simulink model "forerunner_sim_replacement"  (R2016b)
settings: Solver=FixedStepAuto  StartTime=0.0  StopTime=duration  FixedStep=ts  RelTol=1e-3
PreLoadFcn:
  | forerunner_init
undefined symbols (not defined in the file): DiscIntNeverNeededParam, G, G_pitch, G_roll, G_yaw, h, initialEuler, initialPos, LLPV_Filter, P, Q, QC_mpc_rule, qc_update, R, s, S, sd, sdd, t_mpc, tmax, traj_res, UGV_init
libraries: simulink x5
settings Model: sldv_blockreplacement_configurable_lib=forerunner_sim_rt_lib  Creator=Misi  LastModifiedBy=Misi
settings DataIOCC: ReturnWorkspaceOutputs=on
settings DebuggingCC: ArtificialAlgebraicLoopMsg=none
settings SFSimCC: SimUseLocalCustomCode=on
settings RTWCC: RTWUseLocalCustomCode=on

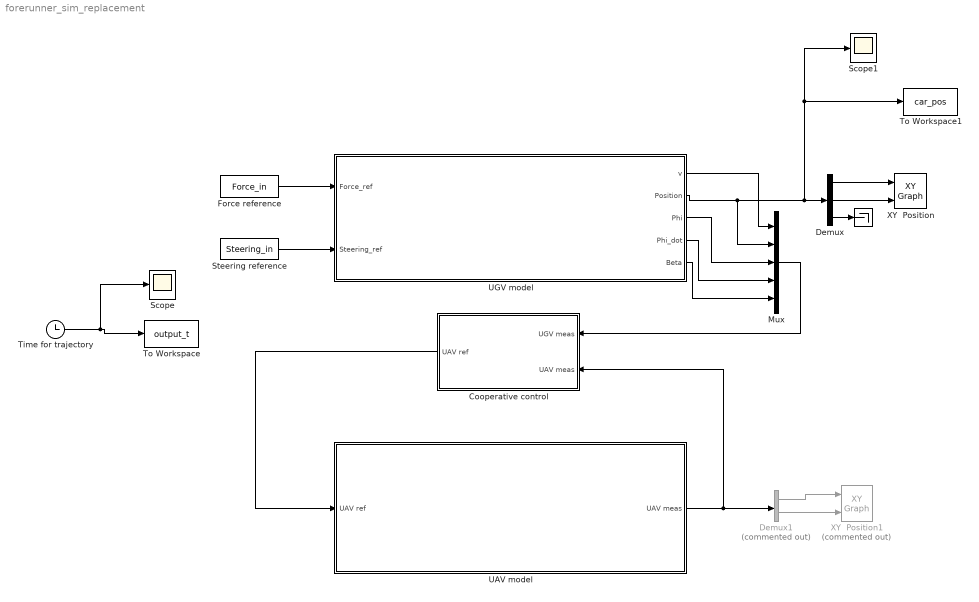
== system forerunner_sim_replacement ==
  " " : Terminator
  Cooperative control : Subsystem
  Demux : Demux  Outputs=3
  Demux1 : Demux  Commented=on  Outputs=2
  "Force reference " : FromWorkspace  VariableName=Force_in  SampleTime=0
  Mux : Mux  Inputs=5
  Scope : Scope
  Scope1 : Scope
  Steering reference : FromWorkspace  VariableName=Steering_in  SampleTime=0
  Time for trajectory : Clock
  To Workspace : ToWorkspace  VariableName=output_t  SampleTime=-1
  To Workspace1 : ToWorkspace  VariableName=car_pos  SampleTime=-1
  UAV model : Subsystem
  UGV model : Subsystem  TreatAsAtomicUnit=on  mask(Sldv ModelReference(Model name:UGV) Replacement){ModelName=UGV, ParameterArgumentNames=, ParameterArgumentValues=, SimulationMode=Normal}
      mask help: Replacement for the Model Reference block that references the model UGV. If Model arguments are specified on the Model Reference block, then they will appear in the mask parameters.
  XY 	Position : simulink/Sinks/XY Graph  xmin=-20  xmax=20  ymin=-20  ymax=20  st=-1
  XY 	Position1 : simulink/Sinks/XY Graph  Commented=on  xmin=-20  xmax=20  ymin=-20  ymax=20  st=-1
  wires:
  "Force reference "/1 -> UGV model/1(Force_ref)
  Steering reference/1 -> UGV model/2(Steering_ref)
  UGV model/2(Position) -> Mux/2, Scope1/1, To Workspace1/1, Demux/1
  Demux/1 -> XY 	Position/1
  Demux/2 -> XY 	Position/2
  UGV model/1(v) -> Mux/1
  UGV model/3(Phi) -> Mux/3
  UGV model/4(Phi_dot) -> Mux/4
  Mux/1 -> Cooperative control/1(UGV meas)
  UAV model/1(UAV meas) -> Cooperative control/2(UAV meas), Demux1/1
  Cooperative control/1(UAV ref) -> UAV model/1(UAV ref)
  Time for trajectory/1 -> Scope/1, To Workspace/1
  Demux/3 -> " "/1
  UGV model/5(Beta) -> Mux/5
  Demux1/1 -> XY 	Position1/1
  Demux1/2 -> XY 	Position1/2

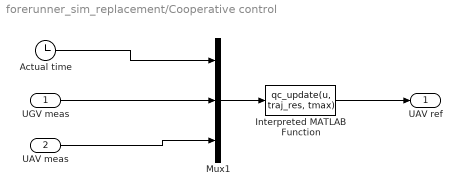
== system forerunner_sim_replacement/Cooperative control ==
  UGV meas : Inport
  UAV meas : Inport  Port=2
  Actual time : Clock
  Interpreted MATLAB Function : MATLABFcn  MATLABFcn=qc_update(u, traj_res, tmax)
  Mux1 : Mux  Inputs=3
  UAV ref : Outport
  wires:
  Interpreted MATLAB Function/1 -> UAV ref/1
  Mux1/1 -> Interpreted MATLAB Function/1
  Actual time/1 -> Mux1/1
  UGV meas/1 -> Mux1/2
  UAV meas/1 -> Mux1/3

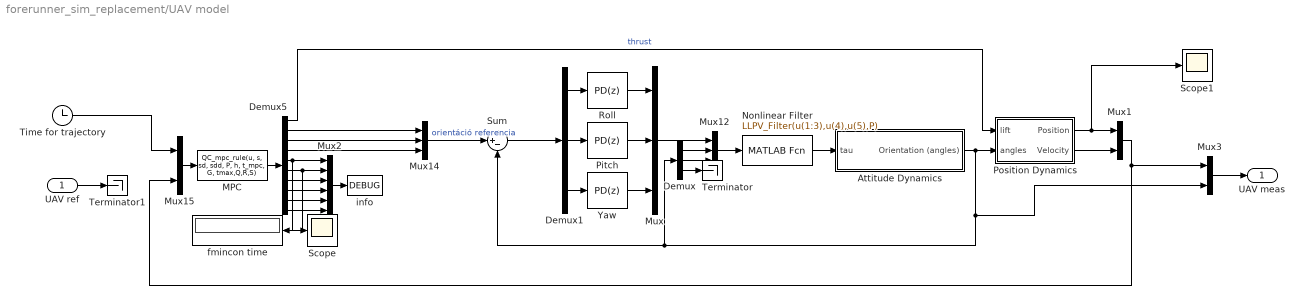
== system forerunner_sim_replacement/UAV model ==
  UAV ref : Inport
  Attitude Dynamics : Subsystem
  Demux : Demux  Outputs=3
  Demux1 : Demux  Outputs=3
  Demux5 : Demux  Outputs=10
  MPC : MATLABFcn  MATLABFcn=QC_mpc_rule(u, s, sd, sdd, P, h, t_mpc, G, tmax,Q,R,S)  OutputDimensions=10
  Mux : Mux  Inputs=3
  Mux1 : Mux  Inputs=2
  Mux12 : Mux  Inputs=3
  Mux14 : Mux  Inputs=3
  Mux15 : Mux  Inputs=2
  Mux2 : Mux  Inputs=6
  Mux3 : Mux  Inputs=2
  Nonlinear Filter : MATLABFcn  MATLABFcn=LLPV_Filter(u(1:3),u(4),u(5),P)  OutputDimensions=3
  Pitch : simulink/Continuous/PID Controller  Controller=PD  TimeDomain=Discrete-time  SampleTime=-1  IntegratorMethod=Forward Euler  FilterMethod=Forward Euler  Form=Parallel  UseFilter=on  ControllerParametersSource=internal  P=G_pitch.Kp  I=1  D=G_pitch.Kd  N=1/G_pitch.Tf  InitialConditionSource=internal  InitialConditionForIntegrator=0  InitialConditionForFilter=0  ExternalReset=none  LimitOutput=off  UpperSaturationLimit=inf  LowerSaturationLimit=-inf  LinearizeAsGain=on  AntiWindupMode=none  Kb=1  TrackingMode=off  Kt=1  PParamMin=[]  PParamMax=[]  IParamMin=[]  IParamMax=[]  DParamMin=[]  DParamMax=[]  NParamMin=[]  NParamMax=[]  KbParamMin=[]  KbParamMax=[]  KtParamMin=[]  KtParamMax=[]  POutMin=[]  POutMax=[]  IOutMin=[]  IOutMax=[]  DOutMin=[]  DOutMax=[]  NOutMin=[]  NOutMax=[]  KbOutMin=[]  KbOutMax=[]  KtOutMin=[]  KtOutMax=[]  IntegratorOutMin=[]  IntegratorOutMax=[]  FilterOutMin=[]  FilterOutMax=[]  SumOutMin=[]  SumOutMax=[]  SumI1OutMin=[]  SumI1OutMax=[]  SumI2OutMin=[]  SumI2OutMax=[]  SumI3OutMin=[]  SumI3OutMax=[]  SumDOutMin=[]  SumDOutMax=[]  SaturationOutMin=[]  SaturationOutMax=[]  IntegratorContinuousStateAttributes=''  IntegratorStateMustResolveToSignalObject=off  IntegratorRTWStateStorageClass=Auto  FilterContinuousStateAttributes=''  FilterStateMustResolveToSignalObject=off  FilterRTWStateStorageClass=Auto  DifferentiatorICPrevScaledInput=0  DifferentiatorOutMin=[]  DifferentiatorOutMax=[]
  Position Dynamics : Subsystem
  Roll : simulink/Continuous/PID Controller  Controller=PD  TimeDomain=Discrete-time  SampleTime=-1  IntegratorMethod=Forward Euler  FilterMethod=Forward Euler  Form=Parallel  UseFilter=on  ControllerParametersSource=internal  P=G_roll.Kp  I=1  D=G_roll.Kd  N=1/G_roll.Tf  InitialConditionSource=internal  InitialConditionForIntegrator=0  InitialConditionForFilter=0  ExternalReset=none  LimitOutput=off  UpperSaturationLimit=inf  LowerSaturationLimit=-inf  LinearizeAsGain=on  AntiWindupMode=none  Kb=1  TrackingMode=off  Kt=1  PParamMin=[]  PParamMax=[]  IParamMin=[]  IParamMax=[]  DParamMin=[]  DParamMax=[]  NParamMin=[]  NParamMax=[]  KbParamMin=[]  KbParamMax=[]  KtParamMin=[]  KtParamMax=[]  POutMin=[]  POutMax=[]  IOutMin=[]  IOutMax=[]  DOutMin=[]  DOutMax=[]  NOutMin=[]  NOutMax=[]  KbOutMin=[]  KbOutMax=[]  KtOutMin=[]  KtOutMax=[]  IntegratorOutMin=[]  IntegratorOutMax=[]  FilterOutMin=[]  FilterOutMax=[]  SumOutMin=[]  SumOutMax=[]  SumI1OutMin=[]  SumI1OutMax=[]  SumI2OutMin=[]  SumI2OutMax=[]  SumI3OutMin=[]  SumI3OutMax=[]  SumDOutMin=[]  SumDOutMax=[]  SaturationOutMin=[]  SaturationOutMax=[]  IntegratorContinuousStateAttributes=''  IntegratorStateMustResolveToSignalObject=off  IntegratorRTWStateStorageClass=Auto  FilterContinuousStateAttributes=''  FilterStateMustResolveToSignalObject=off  FilterRTWStateStorageClass=Auto  DifferentiatorICPrevScaledInput=0  DifferentiatorOutMin=[]  DifferentiatorOutMax=[]
  Scope : Scope
  Scope1 : Scope
  Sum : Sum  Inputs=|+-
  Terminator : Terminator
  Terminator1 : Terminator
  Time for trajectory : Clock
  Yaw : simulink/Continuous/PID Controller  Controller=PD  TimeDomain=Discrete-time  SampleTime=-1  IntegratorMethod=Forward Euler  FilterMethod=Forward Euler  Form=Parallel  UseFilter=on  ControllerParametersSource=internal  P=G_yaw.Kp  I=1  D=G_yaw.Kd  N=1/G_yaw.Tf  InitialConditionSource=internal  InitialConditionForIntegrator=0  InitialConditionForFilter=0  ExternalReset=none  LimitOutput=off  UpperSaturationLimit=inf  LowerSaturationLimit=-inf  LinearizeAsGain=on  AntiWindupMode=none  Kb=1  TrackingMode=off  Kt=1  PParamMin=[]  PParamMax=[]  IParamMin=[]  IParamMax=[]  DParamMin=[]  DParamMax=[]  NParamMin=[]  NParamMax=[]  KbParamMin=[]  KbParamMax=[]  KtParamMin=[]  KtParamMax=[]  POutMin=[]  POutMax=[]  IOutMin=[]  IOutMax=[]  DOutMin=[]  DOutMax=[]  NOutMin=[]  NOutMax=[]  KbOutMin=[]  KbOutMax=[]  KtOutMin=[]  KtOutMax=[]  IntegratorOutMin=[]  IntegratorOutMax=[]  FilterOutMin=[]  FilterOutMax=[]  SumOutMin=[]  SumOutMax=[]  SumI1OutMin=[]  SumI1OutMax=[]  SumI2OutMin=[]  SumI2OutMax=[]  SumI3OutMin=[]  SumI3OutMax=[]  SumDOutMin=[]  SumDOutMax=[]  SaturationOutMin=[]  SaturationOutMax=[]  IntegratorContinuousStateAttributes=''  IntegratorStateMustResolveToSignalObject=off  IntegratorRTWStateStorageClass=Auto  FilterContinuousStateAttributes=''  FilterStateMustResolveToSignalObject=off  FilterRTWStateStorageClass=Auto  DifferentiatorICPrevScaledInput=0  DifferentiatorOutMin=[]  DifferentiatorOutMax=[]
  fmincon time : Display
  info : ToWorkspace  VariableName=DEBUG  SaveFormat=Timeseries  SampleTime=-1
  UAV meas : Outport
  wires:
  Sum/1 -> Demux1/1
  Mux12/1 -> Nonlinear Filter/1
  Mux/1 -> Mux12/1
  Yaw/1 -> Mux/3
  Pitch/1 -> Mux/2
  Roll/1 -> Mux/1
  Demux1/3 -> Yaw/1
  Demux1/2 -> Pitch/1
  Demux1/1 -> Roll/1
  Demux/1 -> Mux12/2
  Demux/2 -> Mux12/3
  Mux14/1 -> Sum/1  "orientáció referencia"
  Mux15/1 -> MPC/1
  Demux/3 -> Terminator/1
  Demux5/1 -> Position Dynamics/1(lift)  "thrust"
  Nonlinear Filter/1 -> Attitude Dynamics/1(tau)
  Mux1/1 -> Mux3/1, Mux15/2
  Time for trajectory/1 -> Mux15/1
  Attitude Dynamics/1(Orientation (angles)) -> Mux3/2, Demux/1, Sum/2, Position Dynamics/2(angles)
  Position Dynamics/1(Position) -> Scope1/1, Mux1/1
  Position Dynamics/2(Velocity) -> Mux1/2
  Demux5/3 -> Mux14/2
  Demux5/4 -> Mux14/3
  MPC/1 -> Demux5/1
  Demux5/5 -> Mux2/1, Scope/1
  Demux5/6 -> fmincon time/1, Mux2/2
  Demux5/7 -> Mux2/3
  Demux5/8 -> Mux2/4
  Demux5/9 -> Mux2/5
  Demux5/10 -> Mux2/6
  Demux5/2 -> Mux14/1
  Mux2/1 -> info/1
  Mux3/1 -> UAV meas/1
  UAV ref/1 -> Terminator1/1

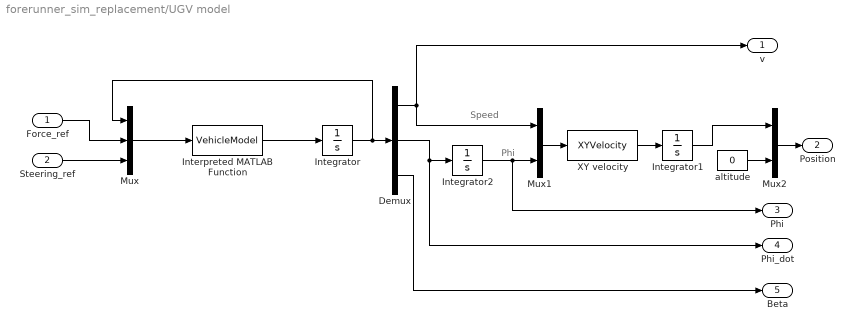
== system forerunner_sim_replacement/UGV model ==
  note: Speed
  note: Phi
  Force_ref : Inport  OutDataTypeStr=double  PortDimensions=1  SampleTime=[0,0]
  Steering_ref : Inport  Port=2  OutDataTypeStr=double  PortDimensions=1  SampleTime=[0,0]
  Demux : Demux  Outputs=3
  Integrator : Integrator  InitialCondition=UGV_init
  Integrator1 : Integrator  InitialCondition=[0 0]
  Integrator2 : Integrator
  Interpreted MATLAB Function : MATLABFcn  MATLABFcn=VehicleModel  OutputDimensions=3
  Mux : Mux  Inputs=3
  Mux1 : Mux  Inputs=2
  Mux2 : Mux  Inputs=2
  XY velocity : MATLABFcn  MATLABFcn=XYVelocity  OutputDimensions=2
  altitude : Constant  Value=0
  v : Outport  OutDataTypeStr=double  PortDimensions=1  SampleTime=[0,0]
  Position : Outport  Port=2  OutDataTypeStr=double  PortDimensions=3
  Phi : Outport  Port=3  OutDataTypeStr=double  PortDimensions=1  SampleTime=[0,0]
  Phi_dot : Outport  Port=4  OutDataTypeStr=double  PortDimensions=1  SampleTime=[0,0]
  Beta : Outport  Port=5  OutDataTypeStr=double  PortDimensions=1  SampleTime=[0,0]
  wires:
  Demux/1 -> v/1, Mux1/1
  altitude/1 -> Mux2/2
  Mux2/1 -> Position/1
  Integrator1/1 -> Mux2/1
  Demux/3 -> Beta/1
  Mux1/1 -> XY velocity/1
  Steering_ref/1 -> Mux/3
  Force_ref/1 -> Mux/2
  XY velocity/1 -> Integrator1/1
  Demux/2 -> Phi_dot/1, Integrator2/1
  Integrator2/1 -> Phi/1, Mux1/2
  Mux/1 -> Interpreted MATLAB Function/1
  Interpreted MATLAB Function/1 -> Integrator/1
  Integrator/1 -> Demux/1, Mux/1

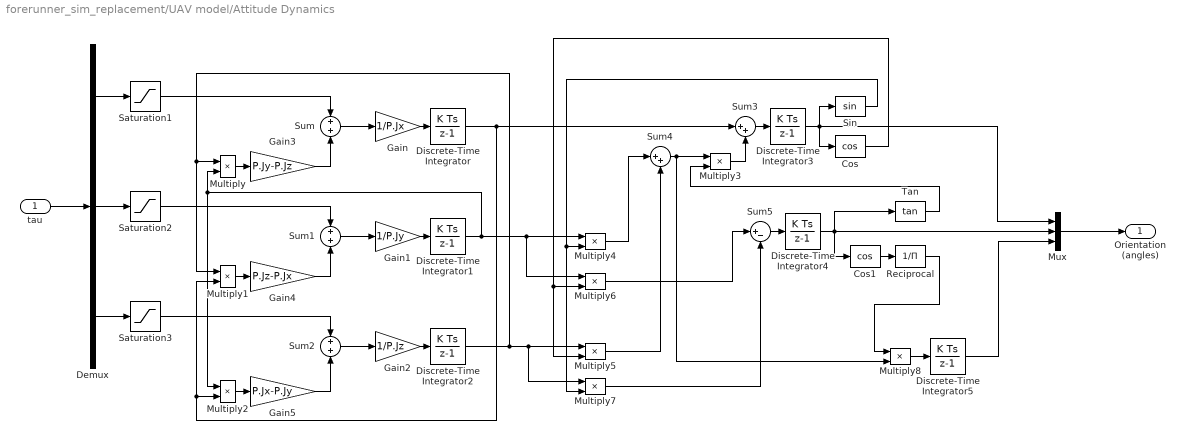
== system forerunner_sim_replacement/UAV model/Attitude Dynamics ==
  tau : Inport
  Cos : Trigonometry  Operator=cos
  Cos1 : Trigonometry  Operator=cos
  Demux : Demux  Outputs=3
  Discrete-Time Integrator : DiscreteIntegrator  InitialCondition=initialEuler(4)  SampleTime=-1  ICPrevOutput=DiscIntNeverNeededParam  ICPrevScaledInput=DiscIntNeverNeededParam
  Discrete-Time Integrator1 : DiscreteIntegrator  InitialCondition=initialEuler(5)  SampleTime=-1  ICPrevOutput=DiscIntNeverNeededParam  ICPrevScaledInput=DiscIntNeverNeededParam
  Discrete-Time Integrator2 : DiscreteIntegrator  InitialCondition=initialEuler(6)  SampleTime=-1  ICPrevOutput=DiscIntNeverNeededParam  ICPrevScaledInput=DiscIntNeverNeededParam
  Discrete-Time Integrator3 : DiscreteIntegrator  InitialCondition=initialEuler(1)  SampleTime=-1  ICPrevOutput=DiscIntNeverNeededParam  ICPrevScaledInput=DiscIntNeverNeededParam
  Discrete-Time Integrator4 : DiscreteIntegrator  InitialCondition=initialEuler(2)  SampleTime=-1  ICPrevOutput=DiscIntNeverNeededParam  ICPrevScaledInput=DiscIntNeverNeededParam
  Discrete-Time Integrator5 : DiscreteIntegrator  InitialCondition=initialEuler(3)  SampleTime=-1  ICPrevOutput=DiscIntNeverNeededParam  ICPrevScaledInput=DiscIntNeverNeededParam
  Gain : Gain  Gain=1/P.Jx
  Gain1 : Gain  Gain=1/P.Jy
  Gain2 : Gain  Gain=1/P.Jz
  Gain3 : Gain  Gain=P.Jy-P.Jz
  Gain4 : Gain  Gain=P.Jz-P.Jx
  Gain5 : Gain  Gain=P.Jx-P.Jy
  Multiply{,1..8} (9 alike) : Product
  Mux : Mux  Inputs=3
  Reciprocal : Product  Inputs=/
  Saturation1 : Saturate  UpperLimit=P.taux  LowerLimit=-P.taux
  Saturation2 : Saturate  UpperLimit=P.tauy  LowerLimit=-P.tauy
  Saturation3 : Saturate  UpperLimit=P.tauz  LowerLimit=-P.tauz
  Sin : Trigonometry
  Sum : Sum
  Sum1 : Sum
  Sum2 : Sum
  Sum3 : Sum  Inputs=|++
  Sum4 : Sum  Inputs=|++
  Sum5 : Sum  Inputs=|+-
  Tan : Trigonometry  Operator=tan
  Orientation (angles) : Outport
  wires:
  tau/1 -> Demux/1
  Discrete-Time Integrator/1 -> Sum3/1, Multiply1/2, Multiply2/2
  Discrete-Time Integrator1/1 -> Multiply4/1, Multiply6/1, Multiply2/1, Multiply/2
  Gain/1 -> Discrete-Time Integrator/1
  Multiply/1 -> Gain3/1
  Multiply1/1 -> Gain4/1
  Multiply2/1 -> Gain5/1
  Gain3/1 -> Sum/2
  Gain4/1 -> Sum1/2
  Gain5/1 -> Sum2/2
  Sum/1 -> Gain/1
  Sum1/1 -> Gain1/1
  Sum2/1 -> Gain2/1
  Discrete-Time Integrator2/1 -> Multiply5/1, Multiply7/1, Multiply1/1, Multiply/1
  Mux/1 -> Orientation (angles)/1
  Discrete-Time Integrator3/1 -> Sin/1, Mux/1, Cos/1
  Discrete-Time Integrator4/1 -> Mux/2, Cos1/1, Tan/1
  Cos1/1 -> Reciprocal/1
  Sum3/1 -> Discrete-Time Integrator3/1
  Multiply3/1 -> Sum3/2
  Cos/1 -> Multiply6/2, Multiply5/2
  Sin/1 -> Multiply7/2, Multiply4/2
  Tan/1 -> Multiply3/2
  Sum4/1 -> Multiply8/2, Multiply3/1
  Multiply4/1 -> Sum4/1
  Multiply5/1 -> Sum4/2
  Sum5/1 -> Discrete-Time Integrator4/1
  Multiply6/1 -> Sum5/1
  Multiply7/1 -> Sum5/2
  Multiply8/1 -> Discrete-Time Integrator5/1
  Reciprocal/1 -> Multiply8/1
  Discrete-Time Integrator5/1 -> Mux/3
  Gain1/1 -> Discrete-Time Integrator1/1
  Gain2/1 -> Discrete-Time Integrator2/1
  Demux/1 -> Saturation1/1
  Demux/3 -> Saturation3/1
  Demux/2 -> Saturation2/1
  Saturation1/1 -> Sum/1
  Saturation2/1 -> Sum1/1
  Saturation3/1 -> Sum2/1

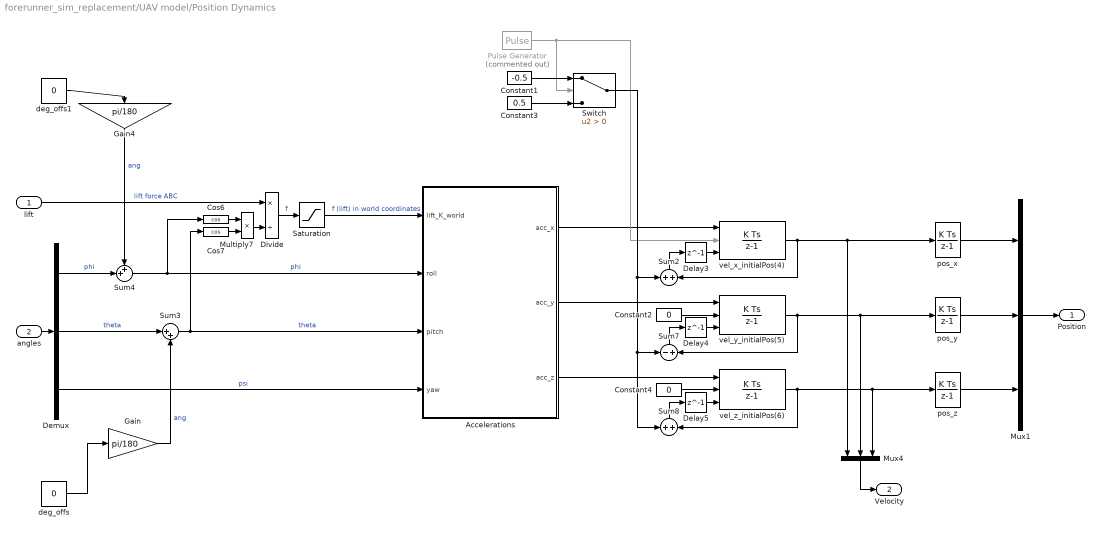
== system forerunner_sim_replacement/UAV model/Position Dynamics ==
  lift : Inport
  angles : Inport  Port=2
  Accelerations : Subsystem
  Constant1 : Constant  Value=-0.5
  Constant2 : Constant  Value=0
  Constant3 : Constant  Value=0.5
  Constant4 : Constant  Value=0
  Cos6 : Trigonometry  Operator=cos
  Cos7 : Trigonometry  Operator=cos
  Delay3 : Delay  DelayLength=1
  Delay4 : Delay  DelayLength=1
  Delay5 : Delay  DelayLength=1
  Demux : Demux  Outputs=3
  Divide : Product  Inputs=*/
  Gain : Gain  Gain=pi/180
  Gain4 : Gain  Gain=pi/180
  Multiply7 : Product
  Mux1 : Mux  Inputs=3
  Mux4 : Mux  Inputs=3
  Pulse Generator : DiscretePulseGenerator  Commented=on  PulseType=Time based  Period=6  PulseWidth=50  PhaseDelay=2
  Saturation : Saturate  UpperLimit=P.Tmax  LowerLimit=0
  Sum2 : Sum  Inputs=+|+
  Sum3 : Sum  Inputs=|++
  Sum4 : Sum  Inputs=++|
  Sum7 : Sum  Inputs=-|+
  Sum8 : Sum  Inputs=+|+
  Switch : Switch  Criteria=u2 > Threshold
  deg_offs : Constant  Value=0
  deg_offs1 : Constant  Value=0
  pos_x : DiscreteIntegrator  InitialCondition=initialPos(1)  SampleTime=-1  ICPrevOutput=DiscIntNeverNeededParam  ICPrevScaledInput=DiscIntNeverNeededParam
  pos_y : DiscreteIntegrator  InitialCondition=initialPos(2)  SampleTime=-1  ICPrevOutput=DiscIntNeverNeededParam  ICPrevScaledInput=DiscIntNeverNeededParam
  pos_z : DiscreteIntegrator  InitialCondition=initialPos(3)  SampleTime=-1  ICPrevOutput=DiscIntNeverNeededParam  ICPrevScaledInput=DiscIntNeverNeededParam
  vel_x_initialPos(4) : DiscreteIntegrator  ExternalReset=either  InitialConditionSource=external  InitialCondition=initialPos(4)  SampleTime=-1  ICPrevOutput=DiscIntNeverNeededParam  ICPrevScaledInput=DiscIntNeverNeededParam
  vel_y_initialPos(5) : DiscreteIntegrator  ExternalReset=falling  InitialConditionSource=external  InitialCondition=initialPos(5)  SampleTime=-1  ICPrevOutput=DiscIntNeverNeededParam  ICPrevScaledInput=DiscIntNeverNeededParam
  vel_z_initialPos(6) : DiscreteIntegrator  ExternalReset=falling  InitialConditionSource=external  InitialCondition=initialPos(6)  SampleTime=-1  ICPrevOutput=DiscIntNeverNeededParam  ICPrevScaledInput=DiscIntNeverNeededParam
  Position : Outport
  Velocity : Outport  Port=2
  wires:
  Sum3/1 -> Cos7/1, Accelerations/3(pitch)  "theta"
  Sum4/1 -> Cos6/1, Accelerations/2(roll)  "phi"
  vel_y_initialPos(5)/1 -> Sum7/2, pos_y/1, Mux4/2
  Accelerations/3(acc_z) -> vel_z_initialPos(6)/1
  Divide/1 -> Saturation/1  "f"
  pos_z/1 -> Mux1/3
  Cos6/1 -> Multiply7/1
  Multiply7/1 -> Divide/2
  Cos7/1 -> Multiply7/2
  lift/1 -> Divide/1  "lift force ABC"
  angles/1 -> Demux/1
  Mux4/1 -> Velocity/1
  Mux1/1 -> Position/1
  Demux/2 -> Sum3/1  "theta"
  deg_offs/1 -> Gain/1
  Gain/1 -> Sum3/2  "ang"
  Demux/1 -> Sum4/2  "phi"
  Gain4/1 -> Sum4/1  "ang"
  deg_offs1/1 -> Gain4/1
  Saturation/1 -> Accelerations/1(lift_K_world)  "f (lift) in world coordinates"
  Demux/3 -> Accelerations/4(yaw)  "psi"
  Accelerations/1(acc_x) -> vel_x_initialPos(4)/1
  Accelerations/2(acc_y) -> vel_y_initialPos(5)/1
  vel_x_initialPos(4)/1 -> Sum2/2, Mux4/1, pos_x/1
  Delay3/1 -> vel_x_initialPos(4)/3
  Sum2/1 -> Delay3/1
  Pulse Generator/1 -> Switch/2, vel_x_initialPos(4)/2
  Sum7/1 -> Delay4/1
  Delay4/1 -> vel_y_initialPos(5)/3
  pos_x/1 -> Mux1/1
  pos_y/1 -> Mux1/2
  vel_z_initialPos(6)/1 -> pos_z/1, Mux4/3, Sum8/2
  Sum8/1 -> Delay5/1
  Delay5/1 -> vel_z_initialPos(6)/3
  Constant2/1 -> vel_y_initialPos(5)/2
  Constant1/1 -> Switch/1
  Constant3/1 -> Switch/3
  Switch/1 -> Sum8/1, Sum7/1, Sum2/1
  Constant4/1 -> vel_z_initialPos(6)/2

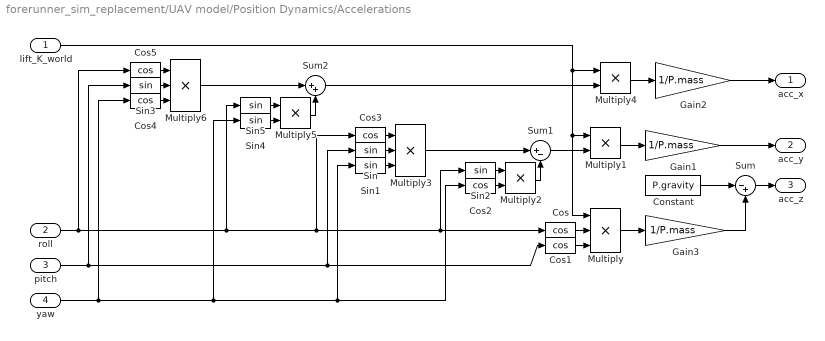
== system forerunner_sim_replacement/UAV model/Position Dynamics/Accelerations ==
  lift_K_world : Inport
  roll : Inport  Port=2
  pitch : Inport  Port=3
  yaw : Inport  Port=4
  Constant : Constant  Value=P.gravity
  Cos{,1..5} (6 alike) : Trigonometry  Operator=cos
  Gain1 : Gain  Gain=1/P.mass
  Gain2 : Gain  Gain=1/P.mass
  Gain3 : Gain  Gain=1/P.mass
  Multiply : Product  Inputs=3
  Multiply{1..2,4..5} (4 alike) : Product
  Multiply3 : Product  Inputs=3
  Multiply6 : Product  Inputs=3
  Sin{,1..5} (6 alike) : Trigonometry
  Sum : Sum  Inputs=|-+
  Sum1 : Sum  Inputs=|+-
  Sum2 : Sum  Inputs=|++
  acc_x : Outport
  acc_y : Outport  Port=2
  acc_z : Outport  Port=3
  wires:
  yaw/1 -> Sin4/1, Sin1/1, Cos2/1, Cos4/1
  Cos2/1 -> Multiply2/2
  Multiply2/1 -> Sum1/2
  Cos1/1 -> Multiply/3
  Sin3/1 -> Multiply6/2
  Gain1/1 -> acc_y/1
  Multiply3/1 -> Sum1/1
  Multiply6/1 -> Sum2/1
  Sum2/1 -> Multiply4/2
  Sum1/1 -> Multiply1/2
  Sin5/1 -> Multiply5/1
  Sin/1 -> Multiply3/2
  Cos/1 -> Multiply/2
  Cos4/1 -> Multiply6/3
  Cos3/1 -> Multiply3/1
  Sin2/1 -> Multiply2/1
  Sin1/1 -> Multiply3/3
  Cos5/1 -> Multiply6/1
  Multiply5/1 -> Sum2/2
  Sin4/1 -> Multiply5/2
  Multiply4/1 -> Gain2/1
  Gain2/1 -> acc_x/1
  Multiply/1 -> Gain3/1
  Multiply1/1 -> Gain1/1
  lift_K_world/1 -> Multiply/1, Multiply1/1, Multiply4/1
  pitch/1 -> Sin3/1, Sin/1, Cos1/1
  roll/1 -> Cos5/1, Cos3/1, Sin2/1, Cos/1, Sin5/1
  Constant/1 -> Sum/1
  Gain3/1 -> Sum/2
  Sum/1 -> acc_z/1
